simulink model "trigger_01"  (R2022a)
settings: Solver=VariableStepAuto  StartTime=0.0  StopTime=10.0  RelTol=1e-3
model workspace (MAT data in the model file):
  out_1 = 0
undefined symbols (not defined in the file): gcbh
settings Model: Creator=FUGAZI  LastModifiedBy=FUGAZI

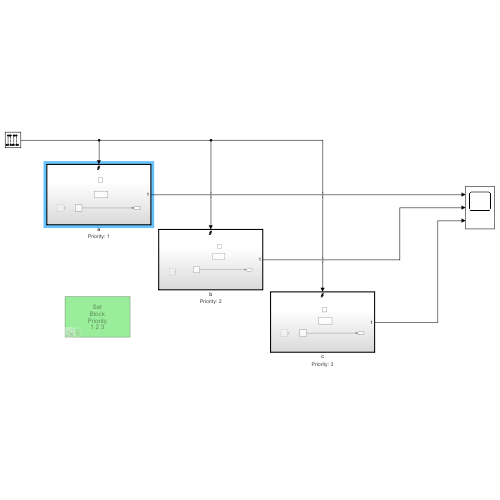
[thumbnail: Simulink's stored preview of the top-level diagram]
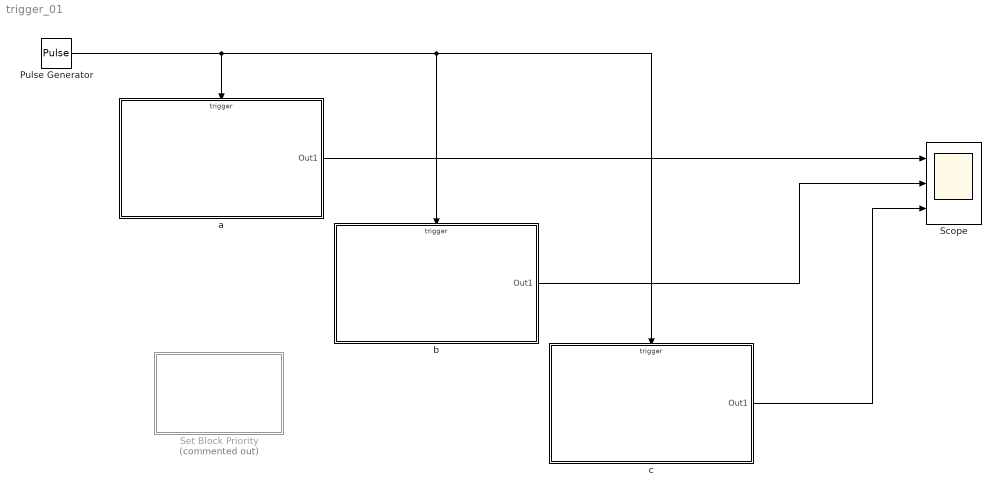
== system trigger_01 ==
  Pulse Generator : DiscretePulseGenerator
  Scope : Scope  NumInputPorts=3
  Set Block Priority : Subsystem  Commented=on  StartFcn=set_param(gcbh,'MaskEnables',{'off'})  StopFcn=set_param(gcbh,'MaskEnables',{'on'})  mask(Set Block Priority){PriorityOrder=1 2 3}
      mask prompts: PriorityOrder "Priority order:"
      mask help: This block lets you select the priority that is used on the three triggered subsystems above it. The priority may only be set when the simulation is stopped.
      mask init:
      | spriorityfcn([],[],[],'PriorityOrder');
      mask TypeOptions PriorityOrder: 1 2 3 | 1 3 2 | 2 1 3 | 2 3 1 | 3 1 2 | 3 2 1
      mask Display: disp(['Set\nBlock\nPriority\n' PriorityOrder])
  a : Subsystem  Priority=1
      settings: AttributesFormatString=Priority: %<Priority>
  b : Subsystem  Priority=2
      settings: AttributesFormatString=Priority: %<Priority>
  c : Subsystem  Priority=3
      settings: AttributesFormatString=Priority: %<Priority>
  wires:
  b/1(Out1) -> Scope/2
  a/1(Out1) -> Scope/1
  c/1(Out1) -> Scope/3
  Pulse Generator/1 -> a/Trigger, b/Trigger, c/Trigger

== system trigger_01/Set Block Priority ==

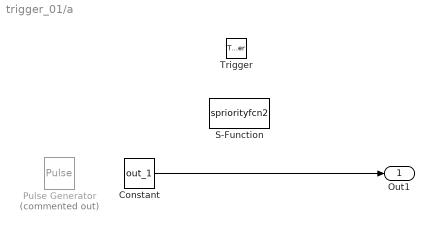
== system trigger_01/a ==
  Trigger : TriggerPort  VariantControl=(inherit)  PortDimensions=1
  Constant : Constant  Value=out_1
  Pulse Generator : DiscretePulseGenerator  Commented=on  PulseType=Time based  PulseWidth=5
  S-Function : S-Function  FunctionName=spriorityfcn2  SFunctionDeploymentMode=off  EnableBusSupport=off
  Out1 : Outport
  wires:
  Constant/1 -> Out1/1

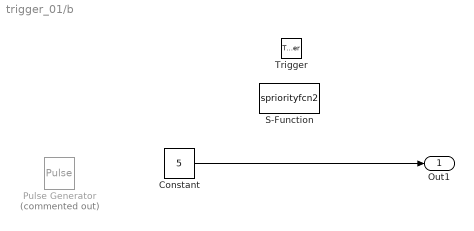
== system trigger_01/b ==
  Trigger : TriggerPort  VariantControl=(inherit)  PortDimensions=1
  Constant : Constant  Value=5
  Pulse Generator : DiscretePulseGenerator  Commented=on  PulseType=Time based  Period=5  PulseWidth=5
  S-Function : S-Function  FunctionName=spriorityfcn2  SFunctionDeploymentMode=off  EnableBusSupport=off
  Out1 : Outport
  wires:
  Constant/1 -> Out1/1

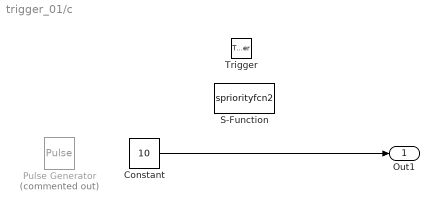
== system trigger_01/c ==
  Trigger : TriggerPort  VariantControl=(inherit)  PortDimensions=1
  Constant : Constant  Value=10
  Pulse Generator : DiscretePulseGenerator  Commented=on  PulseType=Time based  Period=10  PulseWidth=5
  S-Function : S-Function  FunctionName=spriorityfcn2  SFunctionDeploymentMode=off  EnableBusSupport=off
  Out1 : Outport
  wires:
  Constant/1 -> Out1/1
